simulink model "lead_compensator"  (R2018a)
settings: Solver=ode4  StartTime=0.0  StopTime=10.0  FixedStep=0.01  RelTol=1e-3
settings Model: Creator=Kenneth  LastModifiedBy=Kenneth

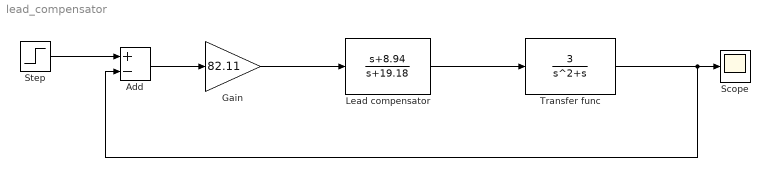
== system lead_compensator ==
  Add : Sum  Inputs=+-
  Gain : Gain  Gain=82.11
  Lead compensator : TransferFcn  Numerator=[1 8.94]  Denominator=[1 19.18]
  Scope : Scope
  Step : Step  Time=0  SampleTime=0
  Transfer func : TransferFcn  Numerator=[3]  Denominator=[1 1 0]
  wires:
  Lead compensator/1 -> Transfer func/1
  Gain/1 -> Lead compensator/1
  Add/1 -> Gain/1
  Step/1 -> Add/1
  Transfer func/1 -> Add/2, Scope/1
